simulink model "ur5_mb1"  (R2024b)
settings: Solver=VariableStepAuto  StartTime=0.0  StopTime=inf  RelTol=1e-3
values from neighbouring files (symbols this model uses):
  N = 500000    [te.m]
undefined symbols (not defined in the file or in its folder): X, Y, Z
libraries: sm_lib x89, nesl_utility x25, sldrtlib x1
(part 3 of 3)

== matlab function ur5_mb1/Subsystem2/MATLAB Function3 ==
  settings: updateMethod=DISCRETE
  data: q_ref output; q_cmd input; t input; A_inc input; A_dec input; Vmax input; w_ref output; pulse input; a_ref output
function [q_ref, w_ref, a_ref] = s_curve_pos_acc(q_cmd, t, A_inc, A_dec, Vmax, pulse)
% q_cmd : 目标位置(rad)
% t     : Clock(s)
% A_inc : 正向(Δq>=0)最大加速度(rad/s^2)
% A_dec : 反向(Δq< 0)最大加速度(rad/s^2)
% Vmax  : 最大速度(rad/s)，不限制就填 Inf
% pulse : 上升沿单脉冲(新指令触发)

persistent q0 v0 a0 qf t0 Tseg c0 c1 c2 c3 c4 c5
if isempty(t0)
    q0 = q_cmd; v0 = 0; a0 = 0;
    qf = q_cmd; t0 = t;
    Tseg = 1e-3;
    [c0,c1,c2,c3,c4,c5] = coeffs(q0,v0,a0,qf,Tseg);
end

% 先按当前段系数算“此刻参考”
[q_now, w_now, a_now] = eval_poly(c0,c1,c2,c3,c4,c5, t - t0, Tseg, qf);

% 触发：锁存新段，并自动算 Tseg
if pulse ~= 0
    q0 = q_now; v0 = w_now; a0 = a_now;
    qf = q_cmd; t0 = t;

    dq = qf - q0;
    if dq >= 0
        Amax = abs(A_inc);
    else
        Amax = abs(A_dec);
    end

    dqabs = abs(dq);
    Tseg = 1e-3;

    if dqabs > 1e-12
        % 对“静止到静止”的五次S曲线：a_peak = (10*sqrt(3)/3) * Δq / T^2
        if Amax > 0
            Tseg = max(Tseg, sqrt((10*sqrt(3)/3) * dqabs / Amax));
        end
        % 可选限速：w_peak = 1.875 * Δq / T
        if isfinite(Vmax) && Vmax > 0
            Tseg = max(Tseg, 1.875 * dqabs / abs(Vmax));
        end

        % 简单迭代：若估计峰值仍超限，就把 Tseg 放大
        for k = 1:4
            [c0,c1,c2,c3,c4,c5] = coeffs(q0,v0,a0,qf,Tseg);
            [v_est, a_est] = estimate_peaks(c0,c1,c2,c3,c4,c5,Tseg);

            scale = 1;
            if isfinite(Vmax) && Vmax > 0
                scale = max(scale, v_est / abs(Vmax));
            end
            if Amax > 0
                scale = max(scale, sqrt(a_est / Amax));
            end

            if scale <= 1.001
                break;
            end
            Tseg = Tseg * scale * 1.05;
        end
    end

    [c0,c1,c2,c3,c4,c5] = coeffs(q0,v0,a0,qf,Tseg);

    % 触发这一拍输出当前值
    q_ref = q0; w_ref = v0; a_ref = a0;
else
    q_ref = q_now; w_ref = w_now; a_ref = a_now;
end
end

function [c0,c1,c2,c3,c4,c5] = coeffs(q0,v0,a0,qf,T)
c0 = q0;
c1 = v0;
c2 = 0.5*a0;

T2 = T*T; T3 = T2*T; T4 = T3*T; T5 = T4*T;

A = qf - (c0 + c1*T + c2*T2);
B = - (c1 + 2*c2*T);   % 终点速度=0
C = - (2*c2);          % 终点加速度=0

c3 = (10*A)/T3 + (-4*B)/T2 + (0.5*C)/T;
c4 = (-15*A)/T4 + (7*B)/T3 + (-C)/T2;
c5 = (6*A)/T5 + (-3*B)/T4 + (0.5*C)/T3;
end

function [q,w,a] = eval_poly(c0,c1,c2,c3,c4,c5,tau,T,qf)
if tau <= 0
    q = c0; w = c1; a = 2*c2; return;
elseif tau >= T
    q = qf; w = 0;  a = 0;  return;
end

t  = tau;
t2 = t*t;  t3 = t2*t;  t4 = t3*t;  t5 = t4*t;

q = c0 + c1*t + c2*t2 + c3*t3 + c4*t4 + c5*t5;
w = c1 + 2*c2*t + 3*c3*t2 + 4*c4*t3 + 5*c5*t4;
a = 2*c2 + 6*c3*t + 12*c4*t2 + 20*c5*t3;
end

function [vmax, amax] = estimate_peaks(c0,c1,c2,c3,c4,c5,T)
vmax = 0; amax = 0;
N = 25;
for i = 0:N
    tau = (T*i)/N;
    [~,w,a] = eval_poly(c0,c1,c2,c3,c4,c5,tau,T,0);
    vmax = max(vmax, abs(w));
    amax = max(amax, abs(a));
end
end

== matlab function ur5_mb1/Subsystem3/MATLAB Function3 ==
  settings: updateMethod=DISCRETE
  data: q_ref output; q_cmd input; t input; A_inc input; A_dec input; Vmax input; w_ref output; pulse input; a_ref output
function [q_ref, w_ref, a_ref] = s_curve_pos_acc(q_cmd, t, A_inc, A_dec, Vmax, pulse)
% q_cmd : 目标位置(rad)
% t     : Clock(s)
% A_inc : 正向(Δq>=0)最大加速度(rad/s^2)
% A_dec : 反向(Δq< 0)最大加速度(rad/s^2)
% Vmax  : 最大速度(rad/s)，不限制就填 Inf
% pulse : 上升沿单脉冲(新指令触发)

persistent q0 v0 a0 qf t0 Tseg c0 c1 c2 c3 c4 c5
if isempty(t0)
    q0 = q_cmd; v0 = 0; a0 = 0;
    qf = q_cmd; t0 = t;
    Tseg = 1e-3;
    [c0,c1,c2,c3,c4,c5] = coeffs(q0,v0,a0,qf,Tseg);
end

% 先按当前段系数算“此刻参考”
[q_now, w_now, a_now] = eval_poly(c0,c1,c2,c3,c4,c5, t - t0, Tseg, qf);

% 触发：锁存新段，并自动算 Tseg
if pulse ~= 0
    q0 = q_now; v0 = w_now; a0 = a_now;
    qf = q_cmd; t0 = t;

    dq = qf - q0;
    if dq >= 0
        Amax = abs(A_inc);
    else
        Amax = abs(A_dec);
    end

    dqabs = abs(dq);
    Tseg = 1e-3;

    if dqabs > 1e-12
        % 对“静止到静止”的五次S曲线：a_peak = (10*sqrt(3)/3) * Δq / T^2
        if Amax > 0
            Tseg = max(Tseg, sqrt((10*sqrt(3)/3) * dqabs / Amax));
        end
        % 可选限速：w_peak = 1.875 * Δq / T
        if isfinite(Vmax) && Vmax > 0
            Tseg = max(Tseg, 1.875 * dqabs / abs(Vmax));
        end

        % 简单迭代：若估计峰值仍超限，就把 Tseg 放大
        for k = 1:4
            [c0,c1,c2,c3,c4,c5] = coeffs(q0,v0,a0,qf,Tseg);
            [v_est, a_est] = estimate_peaks(c0,c1,c2,c3,c4,c5,Tseg);

            scale = 1;
            if isfinite(Vmax) && Vmax > 0
                scale = max(scale, v_est / abs(Vmax));
            end
            if Amax > 0
                scale = max(scale, sqrt(a_est / Amax));
            end

            if scale <= 1.001
                break;
            end
            Tseg = Tseg * scale * 1.05;
        end
    end

    [c0,c1,c2,c3,c4,c5] = coeffs(q0,v0,a0,qf,Tseg);

    % 触发这一拍输出当前值
    q_ref = q0; w_ref = v0; a_ref = a0;
else
    q_ref = q_now; w_ref = w_now; a_ref = a_now;
end
end

function [c0,c1,c2,c3,c4,c5] = coeffs(q0,v0,a0,qf,T)
c0 = q0;
c1 = v0;
c2 = 0.5*a0;

T2 = T*T; T3 = T2*T; T4 = T3*T; T5 = T4*T;

A = qf - (c0 + c1*T + c2*T2);
B = - (c1 + 2*c2*T);   % 终点速度=0
C = - (2*c2);          % 终点加速度=0

c3 = (10*A)/T3 + (-4*B)/T2 + (0.5*C)/T;
c4 = (-15*A)/T4 + (7*B)/T3 + (-C)/T2;
c5 = (6*A)/T5 + (-3*B)/T4 + (0.5*C)/T3;
end

function [q,w,a] = eval_poly(c0,c1,c2,c3,c4,c5,tau,T,qf)
if tau <= 0
    q = c0; w = c1; a = 2*c2; return;
elseif tau >= T
    q = qf; w = 0;  a = 0;  return;
end

t  = tau;
t2 = t*t;  t3 = t2*t;  t4 = t3*t;  t5 = t4*t;

q = c0 + c1*t + c2*t2 + c3*t3 + c4*t4 + c5*t5;
w = c1 + 2*c2*t + 3*c3*t2 + 4*c4*t3 + 5*c5*t4;
a = 2*c2 + 6*c3*t + 12*c4*t2 + 20*c5*t3;
end

function [vmax, amax] = estimate_peaks(c0,c1,c2,c3,c4,c5,T)
vmax = 0; amax = 0;
N = 25;
for i = 0:N
    tau = (T*i)/N;
    [~,w,a] = eval_poly(c0,c1,c2,c3,c4,c5,tau,T,0);
    vmax = max(vmax, abs(w));
    amax = max(amax, abs(a));
end
end

== matlab function ur5_mb1/Triggered Subsystem/MATLAB Function ==
  data: u input; y output; data input
function y = fcn(u, data)

y=0;
if u>0
    y=data;
end
if u<0
    y=-1*data;
end
if u==0
    y=0;
end

== matlab function ur5_mb1/Subsystem1/MATLAB Function3 ==
  settings: updateMethod=DISCRETE
  data: q_ref output; q_cmd input; t input; A_inc input; A_dec input; Vmax input; w_ref output; pulse input; a_ref output
function [q_ref, w_ref, a_ref] = s_curve_pos_acc(q_cmd, t, A_inc, A_dec, Vmax, pulse)
% q_cmd : 目标位置(rad)
% t     : Clock(s)
% A_inc : 正向(Δq>=0)最大加速度(rad/s^2)
% A_dec : 反向(Δq< 0)最大加速度(rad/s^2)
% Vmax  : 最大速度(rad/s)，不限制就填 Inf
% pulse : 上升沿单脉冲(新指令触发)

persistent q0 v0 a0 qf t0 Tseg c0 c1 c2 c3 c4 c5
if isempty(t0)
    q0 = q_cmd; v0 = 0; a0 = 0;
    qf = q_cmd; t0 = t;
    Tseg = 1e-3;
    [c0,c1,c2,c3,c4,c5] = coeffs(q0,v0,a0,qf,Tseg);
end

% 先按当前段系数算“此刻参考”
[q_now, w_now, a_now] = eval_poly(c0,c1,c2,c3,c4,c5, t - t0, Tseg, qf);

% 触发：锁存新段，并自动算 Tseg
if pulse ~= 0
    q0 = q_now; v0 = w_now; a0 = a_now;
    qf = q_cmd; t0 = t;

    dq = qf - q0;
    if dq >= 0
        Amax = abs(A_inc);
    else
        Amax = abs(A_dec);
    end

    dqabs = abs(dq);
    Tseg = 1e-3;

    if dqabs > 1e-12
        % 对“静止到静止”的五次S曲线：a_peak = (10*sqrt(3)/3) * Δq / T^2
        if Amax > 0
            Tseg = max(Tseg, sqrt((10*sqrt(3)/3) * dqabs / Amax));
        end
        % 可选限速：w_peak = 1.875 * Δq / T
        if isfinite(Vmax) && Vmax > 0
            Tseg = max(Tseg, 1.875 * dqabs / abs(Vmax));
        end

        % 简单迭代：若估计峰值仍超限，就把 Tseg 放大
        for k = 1:4
            [c0,c1,c2,c3,c4,c5] = coeffs(q0,v0,a0,qf,Tseg);
            [v_est, a_est] = estimate_peaks(c0,c1,c2,c3,c4,c5,Tseg);

            scale = 1;
            if isfinite(Vmax) && Vmax > 0
                scale = max(scale, v_est / abs(Vmax));
            end
            if Amax > 0
                scale = max(scale, sqrt(a_est / Amax));
            end

            if scale <= 1.001
                break;
            end
            Tseg = Tseg * scale * 1.05;
        end
    end

    [c0,c1,c2,c3,c4,c5] = coeffs(q0,v0,a0,qf,Tseg);

    % 触发这一拍输出当前值
    q_ref = q0; w_ref = v0; a_ref = a0;
else
    q_ref = q_now; w_ref = w_now; a_ref = a_now;
end
end

function [c0,c1,c2,c3,c4,c5] = coeffs(q0,v0,a0,qf,T)
c0 = q0;
c1 = v0;
c2 = 0.5*a0;

T2 = T*T; T3 = T2*T; T4 = T3*T; T5 = T4*T;

A = qf - (c0 + c1*T + c2*T2);
B = - (c1 + 2*c2*T);   % 终点速度=0
C = - (2*c2);          % 终点加速度=0

c3 = (10*A)/T3 + (-4*B)/T2 + (0.5*C)/T;
c4 = (-15*A)/T4 + (7*B)/T3 + (-C)/T2;
c5 = (6*A)/T5 + (-3*B)/T4 + (0.5*C)/T3;
end

function [q,w,a] = eval_poly(c0,c1,c2,c3,c4,c5,tau,T,qf)
if tau <= 0
    q = c0; w = c1; a = 2*c2; return;
elseif tau >= T
    q = qf; w = 0;  a = 0;  return;
end

t  = tau;
t2 = t*t;  t3 = t2*t;  t4 = t3*t;  t5 = t4*t;

q = c0 + c1*t + c2*t2 + c3*t3 + c4*t4 + c5*t5;
w = c1 + 2*c2*t + 3*c3*t2 + 4*c4*t3 + 5*c5*t4;
a = 2*c2 + 6*c3*t + 12*c4*t2 + 20*c5*t3;
end

function [vmax, amax] = estimate_peaks(c0,c1,c2,c3,c4,c5,T)
vmax = 0; amax = 0;
N = 25;
for i = 0:N
    tau = (T*i)/N;
    [~,w,a] = eval_poly(c0,c1,c2,c3,c4,c5,tau,T,0);
    vmax = max(vmax, abs(w));
    amax = max(amax, abs(a));
end
end

== matlab function ur5_mb1/Subsystem4/MATLAB Function3 ==
  settings: updateMethod=DISCRETE
  data: q_ref output; q_cmd input; t input; A_inc input; A_dec input; Vmax input; w_ref output; pulse input; a_ref output
function [q_ref, w_ref, a_ref] = s_curve_pos_acc(q_cmd, t, A_inc, A_dec, Vmax, pulse)
% q_cmd : 目标位置(rad)
% t     : Clock(s)
% A_inc : 正向(Δq>=0)最大加速度(rad/s^2)
% A_dec : 反向(Δq< 0)最大加速度(rad/s^2)
% Vmax  : 最大速度(rad/s)，不限制就填 Inf
% pulse : 上升沿单脉冲(新指令触发)

persistent q0 v0 a0 qf t0 Tseg c0 c1 c2 c3 c4 c5
if isempty(t0)
    q0 = q_cmd; v0 = 0; a0 = 0;
    qf = q_cmd; t0 = t;
    Tseg = 1e-3;
    [c0,c1,c2,c3,c4,c5] = coeffs(q0,v0,a0,qf,Tseg);
end

% 先按当前段系数算“此刻参考”
[q_now, w_now, a_now] = eval_poly(c0,c1,c2,c3,c4,c5, t - t0, Tseg, qf);

% 触发：锁存新段，并自动算 Tseg
if pulse ~= 0
    q0 = q_now; v0 = w_now; a0 = a_now;
    qf = q_cmd; t0 = t;

    dq = qf - q0;
    if dq >= 0
        Amax = abs(A_inc);
    else
        Amax = abs(A_dec);
    end

    dqabs = abs(dq);
    Tseg = 1e-3;

    if dqabs > 1e-12
        % 对“静止到静止”的五次S曲线：a_peak = (10*sqrt(3)/3) * Δq / T^2
        if Amax > 0
            Tseg = max(Tseg, sqrt((10*sqrt(3)/3) * dqabs / Amax));
        end
        % 可选限速：w_peak = 1.875 * Δq / T
        if isfinite(Vmax) && Vmax > 0
            Tseg = max(Tseg, 1.875 * dqabs / abs(Vmax));
        end

        % 简单迭代：若估计峰值仍超限，就把 Tseg 放大
        for k = 1:4
            [c0,c1,c2,c3,c4,c5] = coeffs(q0,v0,a0,qf,Tseg);
            [v_est, a_est] = estimate_peaks(c0,c1,c2,c3,c4,c5,Tseg);

            scale = 1;
            if isfinite(Vmax) && Vmax > 0
                scale = max(scale, v_est / abs(Vmax));
            end
            if Amax > 0
                scale = max(scale, sqrt(a_est / Amax));
            end

            if scale <= 1.001
                break;
            end
            Tseg = Tseg * scale * 1.05;
        end
    end

    [c0,c1,c2,c3,c4,c5] = coeffs(q0,v0,a0,qf,Tseg);

    % 触发这一拍输出当前值
    q_ref = q0; w_ref = v0; a_ref = a0;
else
    q_ref = q_now; w_ref = w_now; a_ref = a_now;
end
end

function [c0,c1,c2,c3,c4,c5] = coeffs(q0,v0,a0,qf,T)
c0 = q0;
c1 = v0;
c2 = 0.5*a0;

T2 = T*T; T3 = T2*T; T4 = T3*T; T5 = T4*T;

A = qf - (c0 + c1*T + c2*T2);
B = - (c1 + 2*c2*T);   % 终点速度=0
C = - (2*c2);          % 终点加速度=0

c3 = (10*A)/T3 + (-4*B)/T2 + (0.5*C)/T;
c4 = (-15*A)/T4 + (7*B)/T3 + (-C)/T2;
c5 = (6*A)/T5 + (-3*B)/T4 + (0.5*C)/T3;
end

function [q,w,a] = eval_poly(c0,c1,c2,c3,c4,c5,tau,T,qf)
if tau <= 0
    q = c0; w = c1; a = 2*c2; return;
elseif tau >= T
    q = qf; w = 0;  a = 0;  return;
end

t  = tau;
t2 = t*t;  t3 = t2*t;  t4 = t3*t;  t5 = t4*t;

q = c0 + c1*t + c2*t2 + c3*t3 + c4*t4 + c5*t5;
w = c1 + 2*c2*t + 3*c3*t2 + 4*c4*t3 + 5*c5*t4;
a = 2*c2 + 6*c3*t + 12*c4*t2 + 20*c5*t3;
end

function [vmax, amax] = estimate_peaks(c0,c1,c2,c3,c4,c5,T)
vmax = 0; amax = 0;
N = 25;
for i = 0:N
    tau = (T*i)/N;
    [~,w,a] = eval_poly(c0,c1,c2,c3,c4,c5,tau,T,0);
    vmax = max(vmax, abs(w));
    amax = max(amax, abs(a));
end
end

== matlab function ur5_mb1/Subsystem5/MATLAB Function3 ==
  settings: updateMethod=DISCRETE
  data: q_ref output; q_cmd input; t input; A_inc input; A_dec input; Vmax input; w_ref output; pulse input; a_ref output
function [q_ref, w_ref, a_ref] = s_curve_pos_acc(q_cmd, t, A_inc, A_dec, Vmax, pulse)
% q_cmd : 目标位置(rad)
% t     : Clock(s)
% A_inc : 正向(Δq>=0)最大加速度(rad/s^2)
% A_dec : 反向(Δq< 0)最大加速度(rad/s^2)
% Vmax  : 最大速度(rad/s)，不限制就填 Inf
% pulse : 上升沿单脉冲(新指令触发)

persistent q0 v0 a0 qf t0 Tseg c0 c1 c2 c3 c4 c5
if isempty(t0)
    q0 = q_cmd; v0 = 0; a0 = 0;
    qf = q_cmd; t0 = t;
    Tseg = 1e-3;
    [c0,c1,c2,c3,c4,c5] = coeffs(q0,v0,a0,qf,Tseg);
end

% 先按当前段系数算“此刻参考”
[q_now, w_now, a_now] = eval_poly(c0,c1,c2,c3,c4,c5, t - t0, Tseg, qf);

% 触发：锁存新段，并自动算 Tseg
if pulse ~= 0
    q0 = q_now; v0 = w_now; a0 = a_now;
    qf = q_cmd; t0 = t;

    dq = qf - q0;
    if dq >= 0
        Amax = abs(A_inc);
    else
        Amax = abs(A_dec);
    end

    dqabs = abs(dq);
    Tseg = 1e-3;

    if dqabs > 1e-12
        % 对“静止到静止”的五次S曲线：a_peak = (10*sqrt(3)/3) * Δq / T^2
        if Amax > 0
            Tseg = max(Tseg, sqrt((10*sqrt(3)/3) * dqabs / Amax));
        end
        % 可选限速：w_peak = 1.875 * Δq / T
        if isfinite(Vmax) && Vmax > 0
            Tseg = max(Tseg, 1.875 * dqabs / abs(Vmax));
        end

        % 简单迭代：若估计峰值仍超限，就把 Tseg 放大
        for k = 1:4
            [c0,c1,c2,c3,c4,c5] = coeffs(q0,v0,a0,qf,Tseg);
            [v_est, a_est] = estimate_peaks(c0,c1,c2,c3,c4,c5,Tseg);

            scale = 1;
            if isfinite(Vmax) && Vmax > 0
                scale = max(scale, v_est / abs(Vmax));
            end
            if Amax > 0
                scale = max(scale, sqrt(a_est / Amax));
            end

            if scale <= 1.001
                break;
            end
            Tseg = Tseg * scale * 1.05;
        end
    end

    [c0,c1,c2,c3,c4,c5] = coeffs(q0,v0,a0,qf,Tseg);

    % 触发这一拍输出当前值
    q_ref = q0; w_ref = v0; a_ref = a0;
else
    q_ref = q_now; w_ref = w_now; a_ref = a_now;
end
end

function [c0,c1,c2,c3,c4,c5] = coeffs(q0,v0,a0,qf,T)
c0 = q0;
c1 = v0;
c2 = 0.5*a0;

T2 = T*T; T3 = T2*T; T4 = T3*T; T5 = T4*T;

A = qf - (c0 + c1*T + c2*T2);
B = - (c1 + 2*c2*T);   % 终点速度=0
C = - (2*c2);          % 终点加速度=0

c3 = (10*A)/T3 + (-4*B)/T2 + (0.5*C)/T;
c4 = (-15*A)/T4 + (7*B)/T3 + (-C)/T2;
c5 = (6*A)/T5 + (-3*B)/T4 + (0.5*C)/T3;
end

function [q,w,a] = eval_poly(c0,c1,c2,c3,c4,c5,tau,T,qf)
if tau <= 0
    q = c0; w = c1; a = 2*c2; return;
elseif tau >= T
    q = qf; w = 0;  a = 0;  return;
end

t  = tau;
t2 = t*t;  t3 = t2*t;  t4 = t3*t;  t5 = t4*t;

q = c0 + c1*t + c2*t2 + c3*t3 + c4*t4 + c5*t5;
w = c1 + 2*c2*t + 3*c3*t2 + 4*c4*t3 + 5*c5*t4;
a = 2*c2 + 6*c3*t + 12*c4*t2 + 20*c5*t3;
end

function [vmax, amax] = estimate_peaks(c0,c1,c2,c3,c4,c5,T)
vmax = 0; amax = 0;
N = 25;
for i = 0:N
    tau = (T*i)/N;
    [~,w,a] = eval_poly(c0,c1,c2,c3,c4,c5,tau,T,0);
    vmax = max(vmax, abs(w));
    amax = max(amax, abs(a));
end
end
